simulink model "CONTROL_JOINT"  (R2019b)
settings: Solver=VariableStepAuto  StartTime=0.0  StopTime=4  RelTol=1e-3
undefined symbols (not defined in the file): axis, K, K_theta, q0, qd0, theta_0, theta_dot_0, time_step
settings Model: Creator=simone  LastModifiedBy=simone

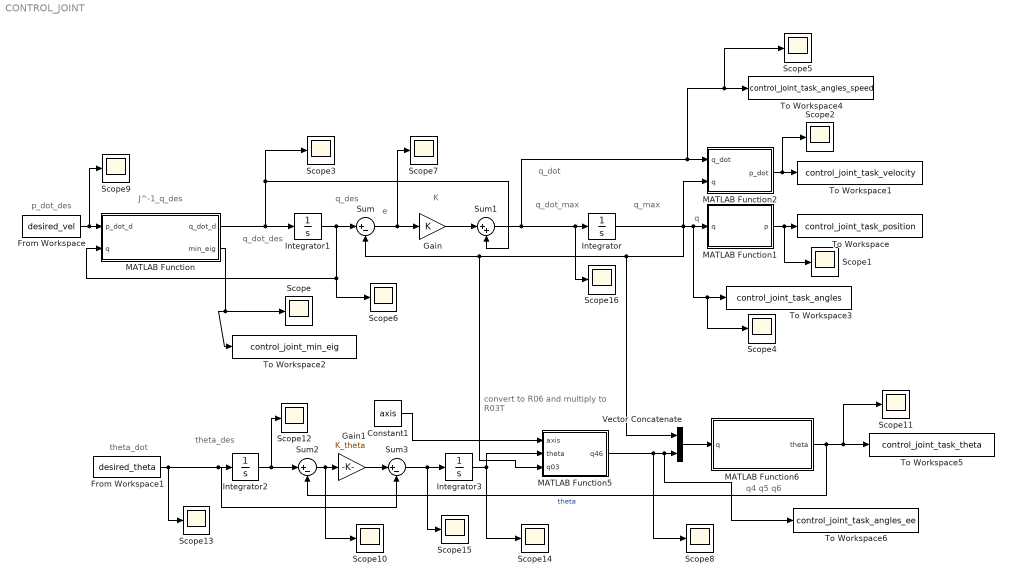
== system CONTROL_JOINT ==
  note: theta_des
  note: q4 q5 q6
  note: convert to R06
      | and multiply to R03T
  note: theta_dot
  note: q_max
  note: q_dot_max
  note: q_dot
  note: q
  note: K
  note: e
  note: q_des
  note: q_dot_des
  note: J^-1_q_des
  note: p_dot_des
  Constant1 : Constant  Value=axis
  From Workspace : FromWorkspace  VariableName=desired_vel  SampleTime=time_step
  From Workspace1 : FromWorkspace  VariableName=desired_theta  SampleTime=time_step
  Gain : Gain  Gain=K
  Gain1 : Gain  Gain=K_theta
  Integrator : Integrator  InitialCondition=q0
  Integrator1 : Integrator  InitialCondition=qd0
  Integrator2 : Integrator  InitialCondition=theta_dot_0
  Integrator3 : Integrator  InitialCondition=theta_0
  MATLAB Function : MATLAB Function  TreatAsAtomicUnit=on
  MATLAB Function1 : MATLAB Function  TreatAsAtomicUnit=on
  MATLAB Function2 : MATLAB Function  TreatAsAtomicUnit=on
  MATLAB Function5 : MATLAB Function  TreatAsAtomicUnit=on
  MATLAB Function6 : MATLAB Function  TreatAsAtomicUnit=on
  Scope{,1..16} (17 alike) : Scope
  Sum : Sum  Inputs=|+-
  Sum1 : Sum  Inputs=|++
  Sum2 : Sum  Inputs=|+-
  Sum3 : Sum  Inputs=|+-
  To Workspace : ToWorkspace  VariableName=control_joint_task_position  SaveFormat=Timeseries  SampleTime=time_step
  To Workspace1 : ToWorkspace  VariableName=control_joint_task_velocity  SaveFormat=Timeseries  SampleTime=time_step
  To Workspace2 : ToWorkspace  VariableName=control_joint_min_eig  SaveFormat=Timeseries  SampleTime=-1
  To Workspace3 : ToWorkspace  VariableName=control_joint_task_angles  SaveFormat=Timeseries  SampleTime=time_step
  To Workspace4 : ToWorkspace  VariableName=control_joint_task_angles_speed  SaveFormat=Timeseries  SampleTime=time_step
  To Workspace5 : ToWorkspace  VariableName=control_joint_task_theta  SaveFormat=Timeseries  SampleTime=time_step
  To Workspace6 : ToWorkspace  VariableName=control_joint_task_angles_ee  SaveFormat=Timeseries  SampleTime=time_step
  Vector Concatenate : Concatenate
  wires:
  From Workspace/1 -> Scope9/1, MATLAB Function/1(p_dot_d)
  MATLAB Function2/1(p_dot) -> To Workspace1/1, Scope2/1
  MATLAB Function1/1(p) -> Scope1/1, To Workspace/1
  Integrator1/1 -> Scope6/1, MATLAB Function/2(q), Sum/1
  Sum/1 -> Scope7/1, Gain/1
  Gain/1 -> Sum1/1
  MATLAB Function/2(min_eig) -> To Workspace2/1, Scope/1
  MATLAB Function/1(q_dot_d) -> Scope3/1, Sum1/2, Integrator1/1
  Sum1/1 -> Scope16/1, Integrator/1, Scope5/1, To Workspace4/1, MATLAB Function2/1(q_dot)
  Constant1/1 -> MATLAB Function5/1(axis)
  Integrator/1 -> Vector Concatenate/1, Sum/2, MATLAB Function5/3(q03), MATLAB Function2/2(q), Scope4/1, To Workspace3/1, MATLAB Function1/1(q)
  From Workspace1/1 -> Scope13/1, Integrator2/1, Sum3/2
  MATLAB Function5/1(q46) -> To Workspace6/1, Vector Concatenate/2, Scope8/1
  Vector Concatenate/1 -> MATLAB Function6/1(q)
  Sum2/1 -> Scope10/1, Gain1/1
  MATLAB Function6/1(theta) -> Scope11/1, To Workspace5/1, Sum2/2  "theta"
  Integrator2/1 -> Scope12/1, Sum2/1
  Gain1/1 -> Sum3/1
  Sum3/1 -> Integrator3/1, Scope15/1
  Integrator3/1 -> Scope14/1, MATLAB Function5/2(theta)

== matlab function CONTROL_JOINT/MATLAB Function1 ==
  data: q input; p output
function p = F_r(q)
% antrophomorphic arm no spherical wrist
%F = [cos(q(1))*(cos(q(2) + q(3)) + cos(q(2))); sin(q(1))*(cos(q(2) + q(3)) + cos(q(2))); sin(q(2) + q(3)) + sin(q(2))];
F = [cos(q(1))*(cos(q(2) + q(3)) + sin(q(2) + q(3)) + cos(q(2))); sin(q(1))*(cos(q(2) + q(3)) + sin(q(2) + q(3)) + cos(q(2))); sin(q(2) + q(3)) - cos(q(2) + q(3)) + sin(q(2))];
p = F;

== matlab function CONTROL_JOINT/MATLAB Function ==
  data: p_dot_d input; q_dot_d output; q input; min_eig output
function [q_dot_d,min_eig] = J_inv_q(p_dot_d,q)
% antrophomorphic arm d3 =1, no d4 (maybe)
% J = [-sin(q(1))*(cos(q(2) + q(3)) + cos(q(2))), -cos(q(1))*(sin(q(2) + q(3)) + sin(q(2))), -sin(q(2) + q(3))*cos(q(1));
%     cos(q(1))*(cos(q(2) + q(3)) + cos(q(2))), -sin(q(1))*(sin(q(2) + q(3)) + sin(q(2))), -sin(q(2) + q(3))*sin(q(1));
%     0, (cos(q(2) + q(3)) + cos(q(2))), cos(q(2) + q(3))];

J = [-sin(q(1))*(cos(q(2)) + sqrt(2)*sin(q(2) + q(3) + pi/4)), -cos(q(1))*(sin(q(2)) - sqrt(2)*cos(q(2) + q(3) + pi/4)), sqrt(2)*cos(q(2) + q(3) + pi/4)*cos(q(1));
    cos(q(1))*(cos(q(2)) + sqrt(2)*sin(q(2) + q(3) + pi/4)), -sin(q(1))*(sin(q(2)) - sqrt(2)*cos(q(2) + q(3) + pi/4)), sqrt(2)*cos(q(2) + q(3) + pi/4)*sin(q(1));
    0, (cos(q(2)) + sqrt(2)*sin(q(2) + q(3) + pi/4)), sqrt(2)*sin(q(2) + q(3) + pi/4)];

min_eig = abs(min(eig(J)));
epsilon_sing = 0.1;

if min_eig < epsilon_sing
    dls_lamb = 0.01;
    J_inv = SR_ROBO.dls_jacobian(J,dls_lamb);
    min_eig = abs(min(eig(J)));
else
    %     J_inv = [-sin(q(1))/(cos(q(2) + q(3)) + cos(q(2))), cos(q(1))/(cos(q(2) + q(3)) + cos(q(2))), 0;
    %         (cos(q(2) + q(3))*cos(q(1)))/sin(q(3)), (cos(q(2) + q(3))*sin(q(1)))/sin(q(3)), sin(q(2) + q(3))/sin(q(3));
    %         -(cos(q(1))*(cos(q(2) + q(3)) + cos(q(2))))/sin(q(3)), -(sin(q(1))*(cos(q(2) + q(3)) + cos(q(2))))/sin(q(3)), -(sin(q(2) + q(3)) + sin(q(2)))/sin(q(3))];
    J_inv = [-(sqrt(2)*sin(q(1)))/(2*sin(q(2) + q(3) + pi/4) + sqrt(2)*cos(q(2))), (sqrt(2)*cos(q(1)))/(2*sin(q(2) + q(3) + pi/4) + sqrt(2)*cos(q(2))), 0;
        -(cos(q(1))*cos(q(2))*cos(q(3)) + cos(q(1))*cos(q(2))*sin(q(3)) + cos(q(1))*cos(q(3))*sin(q(2)) - cos(q(1))*sin(q(2))*sin(q(3)))/(cos(q(3)) - sin(q(3))), -(cos(q(2))*cos(q(3))*sin(q(1)) - sin(q(1))*sin(q(2))*sin(q(3)) + cos(q(2))*sin(q(1))*sin(q(3)) + cos(q(3))*sin(q(1))*sin(q(2)))/(cos(q(3)) - sin(q(3))), cos(q(2) + q(3) + pi/4)/cos(q(3) + pi/4);
        (sqrt(2)*cos(q(1))*(cos(q(2)) + sqrt(2)*sin(q(2) + q(3) + pi/4)))/(2*cos(q(3) + pi/4)), (sqrt(2)*sin(q(1))*(cos(q(2)) + sqrt(2)*sin(q(2) + q(3) + pi/4)))/(2*cos(q(3) + pi/4)), (sqrt(2)*(sin(q(2)) - sqrt(2)*cos(q(2) + q(3) + pi/4)))/(2*cos(q(3) + pi/4))];
    
end


q_dot_d = J_inv*p_dot_d;
end

== matlab function CONTROL_JOINT/MATLAB Function2 ==
  data: q_dot input; p_dot output; q input
function p_dot = J_q(q_dot,q)
% anthropomorphic arm no spherical wrist
% J = [-sin(q(1))*(cos(q(2) + q(3)) + cos(q(2))), -cos(q(1))*(sin(q(2) + q(3)) + sin(q(2))), -sin(q(2) + q(3))*cos(q(1));
%     cos(q(1))*(cos(q(2) + q(3)) + cos(q(2))), -sin(q(1))*(sin(q(2) + q(3)) + sin(q(2))), -sin(q(2) + q(3))*sin(q(1));
%     0, (cos(q(2) + q(3)) + cos(q(2))), cos(q(2) + q(3))];
J = [-sin(q(1))*(cos(q(2)) + sqrt(2)*sin(q(2) + q(3) + pi/4)), -cos(q(1))*(sin(q(2)) - sqrt(2)*cos(q(2) + q(3) + pi/4)), sqrt(2)*cos(q(2) + q(3) + pi/4)*cos(q(1));
    cos(q(1))*(cos(q(2)) + sqrt(2)*sin(q(2) + q(3) + pi/4)), -sin(q(1))*(sin(q(2)) - sqrt(2)*cos(q(2) + q(3) + pi/4)), sqrt(2)*cos(q(2) + q(3) + pi/4)*sin(q(1));
    0, (cos(q(2)) + sqrt(2)*sin(q(2) + q(3) + pi/4)), sqrt(2)*sin(q(2) + q(3) + pi/4)];
p_dot = J*q_dot;

== matlab function CONTROL_JOINT/MATLAB Function5 ==
  data: axis input; q46 output; theta input; q03 input
function q46 = R_zyz(axis,theta, q03)
R06 = axis * axis' + (eye(3,3) - axis * axis') * cos(theta) + [0 -axis(3) axis(2) ; axis(3) 0 -axis(1) ; -axis(2) axis(1) 0 ]*sin(theta);

R03 = [cos(q03(2) + q03(3))*cos(q03(1)), sin(q03(1)), sin(q03(2) + q03(3))*cos(q03(1));
    cos(q03(2) + q03(3))*sin(q03(1)), -cos(q03(1)), sin(q03(2) + q03(3))*sin(q03(1));
    sin(q03(2) + q03(3)), 0, -cos(q03(2) + q03(3))];
R36 = R03' * R06;
q46 = [atan2(R36(2,3),R36(1,3));
    atan2(sqrt(R36(2,3)^2+R36(1,3)^2),R36(3,3));
    atan2(R36(3,2),-R36(3,1))];
end

== matlab function CONTROL_JOINT/MATLAB Function6 ==
  data: q input; theta output
function theta = R_06(q)

R = zeros(3,3);
theta = 0;
R = [sin(q(6))*(cos(q(4))*sin(q(1)) - sin(q(4))*(cos(q(1))*cos(q(2))*cos(q(3)) - cos(q(1))*sin(q(2))*sin(q(3)))) + cos(q(6))*(cos(q(5))*(sin(q(1))*sin(q(4)) + cos(q(4))*(cos(q(1))*cos(q(2))*cos(q(3)) - cos(q(1))*sin(q(2))*sin(q(3)))) - sin(q(5))*(cos(q(1))*cos(q(2))*sin(q(3)) + cos(q(1))*cos(q(3))*sin(q(2)))), cos(q(6))*(cos(q(4))*sin(q(1)) - sin(q(4))*(cos(q(1))*cos(q(2))*cos(q(3)) - cos(q(1))*sin(q(2))*sin(q(3)))) - sin(q(6))*(cos(q(5))*(sin(q(1))*sin(q(4)) + cos(q(4))*(cos(q(1))*cos(q(2))*cos(q(3)) - cos(q(1))*sin(q(2))*sin(q(3)))) - sin(q(5))*(cos(q(1))*cos(q(2))*sin(q(3)) + cos(q(1))*cos(q(3))*sin(q(2)))), sin(q(5))*(sin(q(1))*sin(q(4)) + cos(q(4))*(cos(q(1))*cos(q(2))*cos(q(3)) - cos(q(1))*sin(q(2))*sin(q(3)))) + cos(q(5))*(cos(q(1))*cos(q(2))*sin(q(3)) + cos(q(1))*cos(q(3))*sin(q(2)));
    - sin(q(6))*(cos(q(1))*cos(q(4)) - sin(q(4))*(sin(q(1))*sin(q(2))*sin(q(3)) - cos(q(2))*cos(q(3))*sin(q(1)))) - cos(q(6))*(cos(q(5))*(cos(q(1))*sin(q(4)) + cos(q(4))*(sin(q(1))*sin(q(2))*sin(q(3)) - cos(q(2))*cos(q(3))*sin(q(1)))) + sin(q(5))*(cos(q(2))*sin(q(1))*sin(q(3)) + cos(q(3))*sin(q(1))*sin(q(2)))), sin(q(6))*(cos(q(5))*(cos(q(1))*sin(q(4)) + cos(q(4))*(sin(q(1))*sin(q(2))*sin(q(3)) - cos(q(2))*cos(q(3))*sin(q(1)))) + sin(q(5))*(cos(q(2))*sin(q(1))*sin(q(3)) + cos(q(3))*sin(q(1))*sin(q(2)))) - cos(q(6))*(cos(q(1))*cos(q(4)) - sin(q(4))*(sin(q(1))*sin(q(2))*sin(q(3)) - cos(q(2))*cos(q(3))*sin(q(1)))), cos(q(5))*(cos(q(2))*sin(q(1))*sin(q(3)) + cos(q(3))*sin(q(1))*sin(q(2))) - sin(q(5))*(cos(q(1))*sin(q(4)) + cos(q(4))*(sin(q(1))*sin(q(2))*sin(q(3)) - cos(q(2))*cos(q(3))*sin(q(1))));
    cos(q(6))*(cos(q(2) + q(3))*sin(q(5)) + sin(q(2) + q(3))*cos(q(4))*cos(q(5))) - sin(q(2) + q(3))*sin(q(4))*sin(q(6)), - sin(q(6))*(cos(q(2) + q(3))*sin(q(5)) + sin(q(2) + q(3))*cos(q(4))*cos(q(5))) - sin(q(2) + q(3))*cos(q(6))*sin(q(4)), sin(q(2) + q(3))*cos(q(4))*sin(q(5)) - cos(q(2) + q(3))*cos(q(5))];
axis = zeros(3,1);
theta = atan2(sqrt((R(1,2)-R(2,1))^2+(R(1,3)-R(3,1))^2+(R(2,3)-R(3,2))^2),(R(1,1)+R(2,2)+R(3,3)-1));
if sin(theta) ~= 0
    axis = 1/(2*sin(theta)).*[R(3,2)-R(2,3),R(1,3)-R(3,1),R(2,1)-R(1,2)]';
else
    if abs(theta) == pi
        axis = [sqrt((R(1,1)+1)/2),sqrt((R(2,2)+1)/2),sqrt((R(3,3)+1)/2)]';
    else
        axis = [0 0 0]'; % undefined
    end
end
end
